simulink model "FullCardioLabModel"  (R2023b)
settings: Solver=FixedStepDiscrete  StartTime=0.0  StopTime=param_sim_time  FixedStep=1/fs  MaxStep=1/fs  RelTol=1e-3
undefined symbols (not defined in the file): analyses, fdesignblkfcn, fs, gcbh, param_tot_samples
libraries: dspstat3 x13, SCGAnalysis_SignalGenerationLib x2
(part 1 of 20)
settings Model: PacingRate=100  Creator=rcord  LastModifiedBy=rcord
settings SolverCC: ZeroCrossControl=DisableAll  AlgebraicLoopSolver=TrustRegion
settings DataIOCC: ExternalInput=[t, signals.ecg.input, signals.scg.input_x, signals.scg.input_y, signals.scg.input_z]  LoadExternalInput=on  SignalLogging=off  DSMLogging=off  SaveTime=off  ReturnWorkspaceOutputs=off  TimeSaveName=t_preprocessing  OutputSaveName=out_preprocessing  LoggingIntervals=[-inf,inf]
settings DebuggingCC: UnconnectedInputMsg=warning  UnconnectedOutputMsg=warning  UnconnectedLineMsg=warning
settings ModelReferenceCC: EnableRefExpFcnMdlSchedulingChecks=on
settings SFSimCC: CustomCodeUndefinedFunction=UseInterfaceOnly
settings RTWCC: DLArmComputeVersion=19.05

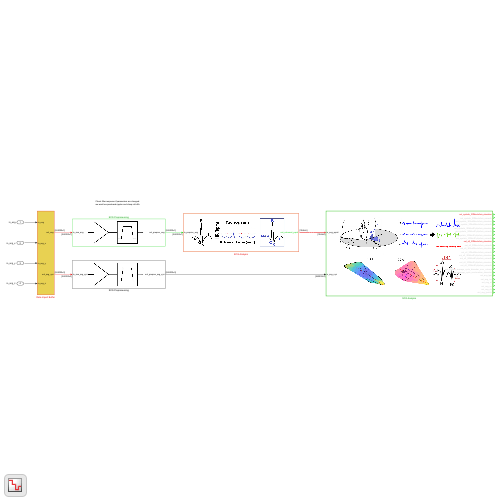
[thumbnail: Simulink's stored preview of the top-level diagram]
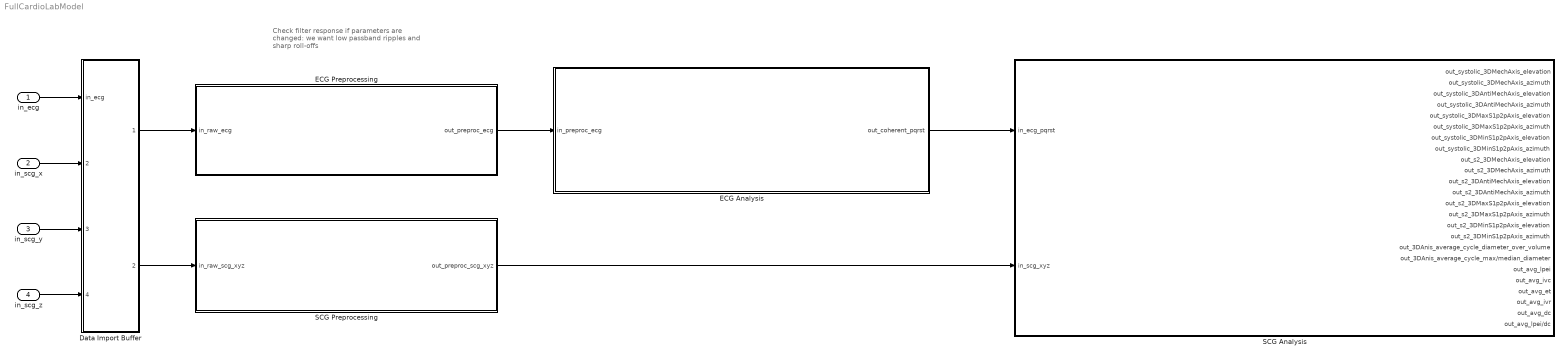
== system FullCardioLabModel ==
  note: Check filter response if parameters are changed:
      | we want low passband ripples and sharp roll-offs
  in_ecg : Inport  SampleTime=1/fs
  in_scg_x : Inport  Port=2  SampleTime=1/fs
  in_scg_y : Inport  Port=3  SampleTime=1/fs
  in_scg_z : Inport  Port=4  SampleTime=1/fs
  Data Import Buffer : Subsystem
  ECG Analysis : Subsystem
      mask Display: image('ECG Analysis2.jpg');
  ECG Preprocessing : Subsystem  mask{param_ecg_gain_mv=1000, param_ecg_fc_lo=1.05, param_ecg_fc_hi=45, param_ecg_trans_bw=1}
      mask prompts: param_ecg_gain_mv "mV Conversion Gain"; param_ecg_fc_lo "Low Passband Frequency Corner (Hz)"; param_ecg_fc_hi "High Passband Frequency Corner (Hz)"; param_ecg_trans_bw "Transition Bandwidth (Hz)"
      mask init:
      | assignin('base','param_ecg_gain_mv',param_ecg_gain_mv)
      | assignin('base','param_ecg_fc_lo',param_ecg_fc_lo)
      | assignin('base','param_ecg_fc_hi',param_ecg_fc_hi)
      | assignin('base','param_ecg_trans_bw',param_ecg_trans_bw)
      mask DialogControl DescGroupVar Prompt: ECG Preprocessing
      mask DialogControl DescTextVar Prompt: Preprocessing stage of the ECG. This involves conversion from V to mV and a filtfilt operation (i.e. a zero-phase FIR filtering) specified by the passband cornerns and transition bandwidth.
      mask Display: image('PreprocessingSymbol.jpg');
  SCG Analysis : Subsystem
      mask Display: image('SCG Analysis.png');
  SCG Preprocessing : Subsystem  mask{param_scg_gain_mg=3333, param_scg_fc_lo=5, param_scg_fc_hi=120, param_scg_trans_bw=2.5}
      mask prompts: param_scg_gain_mg "V to mg Conversion Gain"; param_scg_fc_lo "Low Passband Frequency Corner (Hz)"; param_scg_fc_hi "High Passband Frequency Corner (Hz)"; param_scg_trans_bw "Transition bandwidth"
      mask init:
      | assignin('base','param_scg_gain_mg',param_scg_gain_mg)
      | assignin('base','param_scg_fc_lo',param_scg_fc_lo)
      | assignin('base','param_scg_fc_hi',param_scg_fc_hi)
      | assignin('base','param_scg_trans_bw',param_scg_trans_bw)
      mask DialogControl DescGroupVar Prompt: SCG Preprocessing
      mask DialogControl DescTextVar Prompt: The SCG (x, y, and z) preprocessing block. This involves a V to mg conversion (determined by the transducer sensitivity) and a filtfilt operation. This filtfilt operation consists of a zero-phase FIR front-back filtering that is identical for each of the three cartesian acceleration components and is specified by the passband frequency corners and the transition bandwidth.
      mask Display: image('PreprocessingSymbol.jpg');
  wires:
  in_ecg/1 -> Data Import Buffer/1(in_ecg)
  in_scg_x/1 -> Data Import Buffer/2(in_scg_x)
  in_scg_y/1 -> Data Import Buffer/3(in_scg_y)
  in_scg_z/1 -> Data Import Buffer/4(in_scg_z)
  Data Import Buffer/2(out_scg_xyz) -> SCG Preprocessing/1(in_raw_scg_xyz)
  Data Import Buffer/1(out_ecg) -> ECG Preprocessing/1(in_raw_ecg)
  ECG Preprocessing/1(out_preproc_ecg) -> ECG Analysis/1(in_preproc_ecg)
  SCG Preprocessing/1(out_preproc_scg_xyz) -> SCG Analysis/2(in_scg_xyz)
  ECG Analysis/1(out_coherent_pqrst) -> SCG Analysis/1(in_ecg_pqrst)

== system FullCardioLabModel/Data Import Buffer ==
  in_ecg : Inport
  in_scg_x : Inport  Port=2
  in_scg_y : Inport  Port=3
  in_scg_z : Inport  Port=4
  Buffer{,1..3} (4 alike) : Buffer  N=param_tot_samples  OutputFrames=off
  Vector Concatenate : Concatenate  NumInputs=3  Mode=Multidimensional array  ConcatenateDimension=2
  out_ecg : Outport  VectorParamsAs1DForOutWhenUnconnected=off
  out_scg_xyz : Outport  Port=2  VectorParamsAs1DForOutWhenUnconnected=off
  wires:
  in_ecg/1 -> Buffer1/1
  Buffer/1 -> Vector Concatenate/3  "scg_z"
  Buffer3/1 -> Vector Concatenate/1  "scg_x"
  in_scg_x/1 -> Buffer3/1
  Vector Concatenate/1 -> out_scg_xyz/1
  Buffer1/1 -> out_ecg/1
  Buffer2/1 -> Vector Concatenate/2  "scg_y"
  in_scg_z/1 -> Buffer/1
  in_scg_y/1 -> Buffer2/1

== system FullCardioLabModel/ECG Analysis ==
  in_preproc_ecg : Inport
  Enabled ECG Analysis Subsystem : Subsystem  TreatAsAtomicUnit=on
  out_coherent_pqrst : Outport
  wires:
  in_preproc_ecg/1 -> Enabled ECG Analysis Subsystem/Enable
  Enabled ECG Analysis Subsystem/1(idxs_coherent_pqrst) -> out_coherent_pqrst/1

== system FullCardioLabModel/ECG Preprocessing ==
  in_raw_ecg : Inport
  Enabled ECG Preprocessing Subsystem : Subsystem  TreatAsAtomicUnit=on
  out_preproc_ecg : Outport  VectorParamsAs1DForOutWhenUnconnected=off
  wires:
  Enabled ECG Preprocessing Subsystem/1(Output) -> out_preproc_ecg/1
  in_raw_ecg/1 -> Enabled ECG Preprocessing Subsystem/Enable

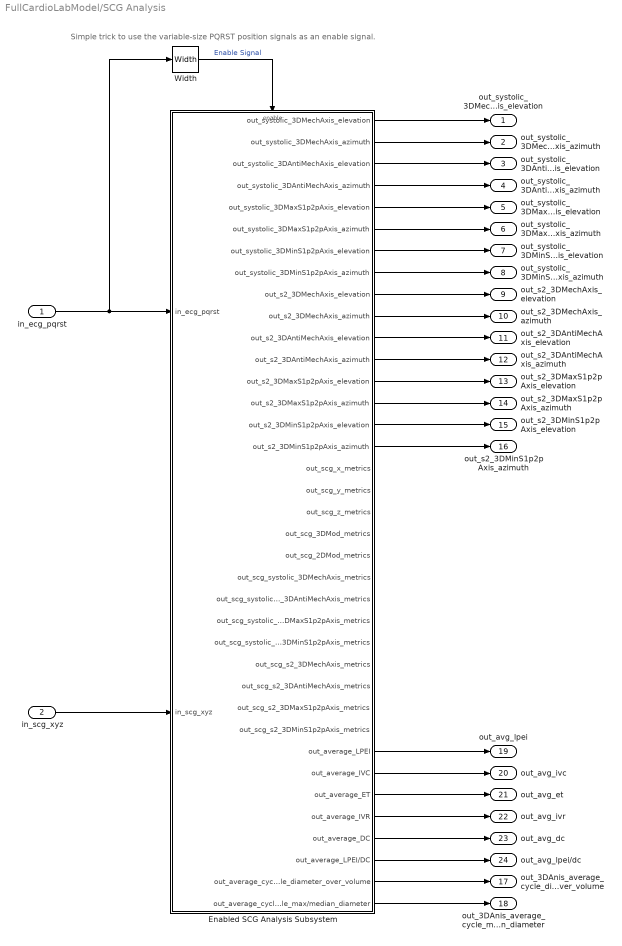
== system FullCardioLabModel/SCG Analysis ==
  note: Simple trick to use the variable-size PQRST position signals as an enable signal.
  in_ecg_pqrst : Inport
  in_scg_xyz : Inport  Port=2
  Enabled SCG Analysis Subsystem : Subsystem  TreatAsAtomicUnit=on
  "Width " : Width
  out_systolic_3DMechAxis_elevation : Outport  VectorParamsAs1DForOutWhenUnconnected=off
  out_systolic_3DMechAxis_azimuth : Outport  Port=2  VectorParamsAs1DForOutWhenUnconnected=off
  out_systolic_3DAntiMechAxis_elevation : Outport  Port=3  VectorParamsAs1DForOutWhenUnconnected=off
  out_systolic_3DAntiMechAxis_azimuth : Outport  Port=4  VectorParamsAs1DForOutWhenUnconnected=off
  out_systolic_3DMaxS1p2pAxis_elevation : Outport  Port=5  VectorParamsAs1DForOutWhenUnconnected=off
  out_systolic_3DMaxS1p2pAxis_azimuth : Outport  Port=6  VectorParamsAs1DForOutWhenUnconnected=off
  out_systolic_3DMinS1p2pAxis_elevation : Outport  Port=7  VectorParamsAs1DForOutWhenUnconnected=off
  out_systolic_3DMinS1p2pAxis_azimuth : Outport  Port=8  VectorParamsAs1DForOutWhenUnconnected=off
  out_s2_3DMechAxis_elevation : Outport  Port=9  VectorParamsAs1DForOutWhenUnconnected=off
  out_s2_3DMechAxis_azimuth : Outport  Port=10  VectorParamsAs1DForOutWhenUnconnected=off
  out_s2_3DAntiMechAxis_elevation : Outport  Port=11  VectorParamsAs1DForOutWhenUnconnected=off
  out_s2_3DAntiMechAxis_azimuth : Outport  Port=12  VectorParamsAs1DForOutWhenUnconnected=off
  out_s2_3DMaxS1p2pAxis_elevation : Outport  Port=13  VectorParamsAs1DForOutWhenUnconnected=off
  out_s2_3DMaxS1p2pAxis_azimuth : Outport  Port=14  VectorParamsAs1DForOutWhenUnconnected=off
  out_s2_3DMinS1p2pAxis_elevation : Outport  Port=15  VectorParamsAs1DForOutWhenUnconnected=off
  out_s2_3DMinS1p2pAxis_azimuth : Outport  Port=16  VectorParamsAs1DForOutWhenUnconnected=off
  out_3DAnis_average_cycle_diameter_over_volume : Outport  Port=17  VectorParamsAs1DForOutWhenUnconnected=off
  out_3DAnis_average_cycle_max/median_diameter : Outport  Port=18  VectorParamsAs1DForOutWhenUnconnected=off
  out_avg_lpei : Outport  Port=19  VectorParamsAs1DForOutWhenUnconnected=off
  out_avg_ivc : Outport  Port=20  VectorParamsAs1DForOutWhenUnconnected=off
  out_avg_et : Outport  Port=21  VectorParamsAs1DForOutWhenUnconnected=off
  out_avg_ivr : Outport  Port=22  VectorParamsAs1DForOutWhenUnconnected=off
  out_avg_dc : Outport  Port=23  VectorParamsAs1DForOutWhenUnconnected=off
  out_avg_lpei/dc : Outport  Port=24  VectorParamsAs1DForOutWhenUnconnected=off
  wires:
  in_scg_xyz/1 -> Enabled SCG Analysis Subsystem/2(in_scg_xyz)
  in_ecg_pqrst/1 -> "Width "/1, Enabled SCG Analysis Subsystem/1(in_ecg_pqrst)
  "Width "/1 -> Enabled SCG Analysis Subsystem/Enable  "Enable Signal"
  Enabled SCG Analysis Subsystem/1(out_systolic_3DMechAxis_elevation) -> out_systolic_3DMechAxis_elevation/1
  Enabled SCG Analysis Subsystem/2(out_systolic_3DMechAxis_azimuth) -> out_systolic_3DMechAxis_azimuth/1
  Enabled SCG Analysis Subsystem/8(out_systolic_3DMinS1p2pAxis_azimuth) -> out_systolic_3DMinS1p2pAxis_azimuth/1
  Enabled SCG Analysis Subsystem/7(out_systolic_3DMinS1p2pAxis_elevation) -> out_systolic_3DMinS1p2pAxis_elevation/1
  Enabled SCG Analysis Subsystem/6(out_systolic_3DMaxS1p2pAxis_azimuth) -> out_systolic_3DMaxS1p2pAxis_azimuth/1
  Enabled SCG Analysis Subsystem/5(out_systolic_3DMaxS1p2pAxis_elevation) -> out_systolic_3DMaxS1p2pAxis_elevation/1
  Enabled SCG Analysis Subsystem/4(out_systolic_3DAntiMechAxis_azimuth) -> out_systolic_3DAntiMechAxis_azimuth/1
  Enabled SCG Analysis Subsystem/3(out_systolic_3DAntiMechAxis_elevation) -> out_systolic_3DAntiMechAxis_elevation/1
  Enabled SCG Analysis Subsystem/37(out_average_cycle_cycle_max/median_diameter) -> out_3DAnis_average_cycle_max/median_diameter/1
  Enabled SCG Analysis Subsystem/36(out_average_cycle_diameter_over_volume) -> out_3DAnis_average_cycle_diameter_over_volume/1
  Enabled SCG Analysis Subsystem/12(out_s2_3DAntiMechAxis_azimuth) -> out_s2_3DAntiMechAxis_azimuth/1
  Enabled SCG Analysis Subsystem/10(out_s2_3DMechAxis_azimuth) -> out_s2_3DMechAxis_azimuth/1
  Enabled SCG Analysis Subsystem/13(out_s2_3DMaxS1p2pAxis_elevation) -> out_s2_3DMaxS1p2pAxis_elevation/1
  Enabled SCG Analysis Subsystem/11(out_s2_3DAntiMechAxis_elevation) -> out_s2_3DAntiMechAxis_elevation/1
  Enabled SCG Analysis Subsystem/14(out_s2_3DMaxS1p2pAxis_azimuth) -> out_s2_3DMaxS1p2pAxis_azimuth/1
  Enabled SCG Analysis Subsystem/15(out_s2_3DMinS1p2pAxis_elevation) -> out_s2_3DMinS1p2pAxis_elevation/1
  Enabled SCG Analysis Subsystem/16(out_s2_3DMinS1p2pAxis_azimuth) -> out_s2_3DMinS1p2pAxis_azimuth/1
  Enabled SCG Analysis Subsystem/9(out_s2_3DMechAxis_elevation) -> out_s2_3DMechAxis_elevation/1
  Enabled SCG Analysis Subsystem/30(out_average_LPEI) -> out_avg_lpei/1
  Enabled SCG Analysis Subsystem/31(out_average_IVC) -> out_avg_ivc/1
  Enabled SCG Analysis Subsystem/32(out_average_ET) -> out_avg_et/1
  Enabled SCG Analysis Subsystem/33(out_average_IVR) -> out_avg_ivr/1
  Enabled SCG Analysis Subsystem/34(out_average_DC) -> out_avg_dc/1
  Enabled SCG Analysis Subsystem/35(out_average_LPEI/DC) -> out_avg_lpei/dc/1

== system FullCardioLabModel/SCG Preprocessing ==
  in_raw_scg_xyz : Inport
  Enabled SCG Preprocessing Subsystem : Subsystem  TreatAsAtomicUnit=on
  out_preproc_scg_xyz : Outport  VectorParamsAs1DForOutWhenUnconnected=off
  wires:
  Enabled SCG Preprocessing Subsystem/1(out_preprocessed_scg_xyz) -> out_preproc_scg_xyz/1
  in_raw_scg_xyz/1 -> Enabled SCG Preprocessing Subsystem/Enable

== system FullCardioLabModel/ECG Analysis/Enabled ECG Analysis Subsystem ==
  note: The subsystem is only enabled when it receives a (non-zero) signal
  Preprocessed ECG : EnablePort  PropagateVarSize=During execution  ShowOutputPort=on
  Assign To Workspace: Num Cycles : Subsystem
      mask Display: disp('Assign: out_ecg_num_cycles')
  Assign To Workspace: idxs PQRST : Subsystem
      mask Display: disp('Assign: out_idxs_pqrst')
  Coherent Segmentation : Subsystem
      mask Display: image('Coherent ECG.jpg');
  Constant : Constant  Value=fs
  Ectopic Correction : Subsystem  mask{max_hr=200, max_hr_dev=40}
      mask prompts: max_hr "Maximum Heart Rate (in bpm)"; max_hr_dev "Maximum HR Deviation (in bpm)"
      mask DialogControl DescGroupVar Prompt: Ectopic Correction
      mask DialogControl DescTextVar Prompt: Specify the ectopic detection parameters. What will be defined as an ectopic cycle and removed from further analysis? Maximum heart rate specifies the upper limit of heart rate - any cycles with RR intervals corresponding to heart rates above this limit will be considered ectopic. Maximum HR deviation - any cycles with an instantaneous HR greater than this deviation from the moving average HR will be considered ectopic.
      mask Display: image('Tachogram.jpg');
  Labelled ECG Plotting : MATLAB Function  TreatAsAtomicUnit=on
  Num Cycles : Display
  P,Q,R,S,T Detection : Subsystem  mask{ecg_algo=PQRST waves - Multi-level Teager Energy Operator}
      mask prompts: ecg_algo "Choose one:"
      mask init:
      | if ecg_algo == 1
      |     param_ecg_algo = 'Pan-Tompkins';
      | elseif ecg_algo == 2
      |     param_ecg_algo = 'Phase Space';
      | elseif ecg_algo == 3
      |     param_ecg_algo = 'Filter Bank';
      | elseif ecg_algo == 4
      |     param_ecg_algo = 'State Machine';
      | elseif ecg_algo == 5
      |     param_ecg_algo = 'Multi-level Teager Energy Operator';
      | end
      | 
      | assignin('base','param_ecg_algo', param_ecg_algo)
      mask TypeOptions ecg_algo: R wave  - Pan-Tompkins | R wave - Phase space | R wave - Filter bank | QRST waves - State machine | PQRST waves - Multi-level Teager Energy Operator
      mask DialogControl DescGroupVar Prompt: ECG PQRST Detection
      mask DialogControl DescTextVar Prompt: Select detected waveform(s) and corresponding detection aglorithm.
      mask DialogControl ParameterGroupVar Prompt: Desired wave(s) and Algorithm
      mask Display: image('Labelled ECG2.jpg');
  idxs_coherent_pqrst : Outport
  wires:
  Preprocessed ECG/1 -> P,Q,R,S,T Detection/1(Preprocessed ECG), Labelled ECG Plotting/2(preprocessed_ecg)
  P,Q,R,S,T Detection/3(idxs_r) -> Ectopic Correction/1(r_pos)
  Constant/1 -> Labelled ECG Plotting/3(fs)
  Coherent Segmentation/2(num_cycles) -> Assign To Workspace: Num Cycles/1(In1), Num Cycles/1
  Ectopic Correction/1(corrected_r_pos) -> Coherent Segmentation/3(idxs_r)
  Coherent Segmentation/1(idxs_coherent_pqrst) -> Assign To Workspace: idxs PQRST/1(in_idxs_pqrst), idxs_coherent_pqrst/1, Labelled ECG Plotting/1(idxs_coherent_pqrst)
  P,Q,R,S,T Detection/5(idxs_t) -> Coherent Segmentation/5(idxs_t)
  P,Q,R,S,T Detection/4(idxs_s) -> Coherent Segmentation/4(idxs_s)
  P,Q,R,S,T Detection/1(idxs_p) -> Coherent Segmentation/1(idxs_p)
  P,Q,R,S,T Detection/2(idxs_q) -> Coherent Segmentation/2(idxs_q)

== system FullCardioLabModel/ECG Preprocessing/Enabled ECG Preprocessing Subsystem ==
  note: The subsystem is only enabled when it receives a (non-zero) signal
  in_ecg : EnablePort  ShowOutputPort=on
  Constant : Constant  Value=fs
  ECG Filtfiltering : Subsystem
  ECG Preprocessing Input (Frequency) : SpectrumAnalyzer  Commented=on  WindowPosition=[1 1 1312 537]  Method=Welch  SampleRate=1000  PlotAsTwoSidedSpectrum=off  Span=500  CenterFrequency=250  StartFrequency=0  StopFrequency=500  FrequencyResolutionMethod=Window length  WindowLength=param_tot_samples/10  Window=Rectangular  AveragingMethod=Running  SpectralAverages=10  YLimits=[-135.30878679633289607,-53.597859807423823497]  ShowLegend=on  DefaultConfigurationName=spbscopes.SpectrumAnalyzerBlockCfg  IsFrequencyInputMode=0  FrequencyVectorPort=0  FrequencyVectorFromPort=0  FrequencyInputRBWPort=0  FrequencyInputRBWFromPort=0
  ECG Preprocessing Input (Time) : Scope  Commented=on
  ECG Preprocessing Output (Frequency) : SpectrumAnalyzer  Commented=on  WindowPosition=[1 1 1312 537]  Method=Welch  SampleRateSource=Property  SampleRate=1/fs  PlotAsTwoSidedSpectrum=off  Span=0.0005  CenterFrequency=0.00025  StartFrequency=0  StopFrequency=0.0005  FrequencyResolutionMethod=Window length  WindowLength=param_tot_samples/10  Window=Rectangular  AveragingMethod=Running  SpectralAverages=10  YLimits=[-88.467038023731845442,-3.7161177694563978235]  ShowLegend=on  DefaultConfigurationName=spbscopes.SpectrumAnalyzerBlockCfg  IsFrequencyInputMode=0  FrequencyVectorPort=0  FrequencyVectorFromPort=0  FrequencyInputRBWPort=0  FrequencyInputRBWFromPort=0
  ECG Preprocessing Output (Time) : Scope
  Plotting : MATLAB Function  TreatAsAtomicUnit=on
  To Workspace: Processed ECG : Subsystem
      mask Display: disp('out_ecg_preprocessing')
  V to mV Conversion : Gain  Gain=param_ecg_gain_mv
  Output : Outport  VectorParamsAs1DForOutWhenUnconnected=off
  wires:
  V to mV Conversion/1 -> ECG Filtfiltering/1(input ecg)
  in_ecg/1 -> V to mV Conversion/1, ECG Preprocessing Input (Time)/1, Plotting/2(raw_ecg), ECG Preprocessing Input (Frequency)/1
  ECG Filtfiltering/1(filtfiltered ecg) -> To Workspace: Processed ECG/1(In1), Output/1, ECG Preprocessing Output (Time)/1, Plotting/1(preprocessed_ecg), ECG Preprocessing Output (Frequency)/1
  Constant/1 -> Plotting/3(fs)

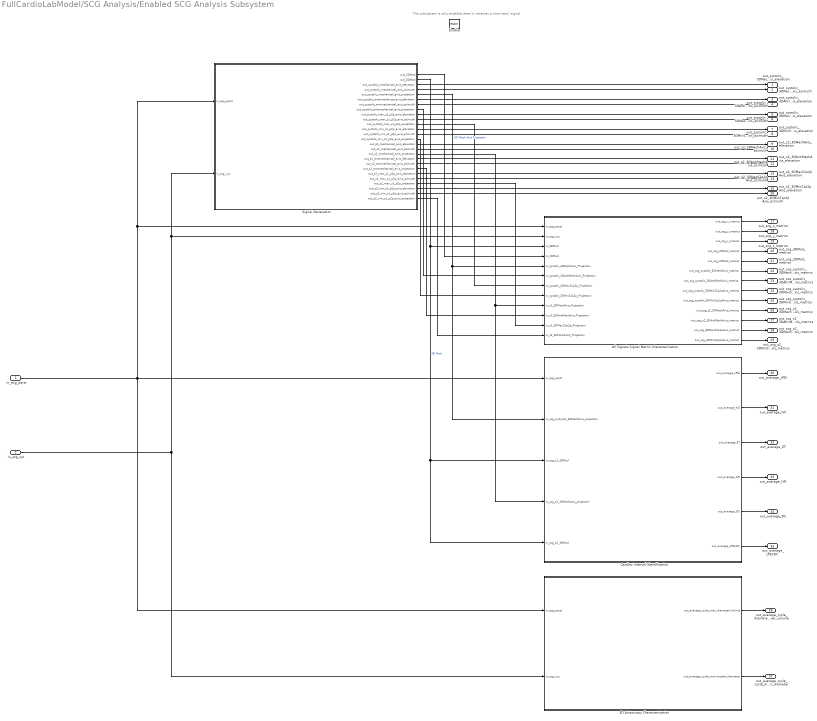
== system FullCardioLabModel/SCG Analysis/Enabled SCG Analysis Subsystem ==
  note: The subsystem is only enabled when it receives a (non-zero) signal
  in_ecg_pqrst : Inport
  in_scg_xyz : Inport  Port=2
  Enable : EnablePort  StatesWhenEnabling=reset  PropagateVarSize=During execution
  3D Anisotropy Characterization : Subsystem
      mask Display: image('Anisotropy.png');
  All Signals Signal Metric Characterization : Subsystem
      mask Display: image('Characterization.png');
  Cardiac Interval Identification : Subsystem
      mask Display: image('Systolic Intervals.png');
  Signal Generation : Subsystem
      mask Display: image('Signal Generation.png');
  out_systolic_3DMechAxis_elevation : Outport  VectorParamsAs1DForOutWhenUnconnected=off
  out_systolic_3DMechAxis_azimuth : Outport  Port=2  VectorParamsAs1DForOutWhenUnconnected=off
  out_systolic_3DAntiMechAxis_elevation : Outport  Port=3  VectorParamsAs1DForOutWhenUnconnected=off
  out_systolic_3DAntiMechAxis_azimuth : Outport  Port=4  VectorParamsAs1DForOutWhenUnconnected=off
  out_systolic_3DMaxS1p2pAxis_elevation : Outport  Port=5  VectorParamsAs1DForOutWhenUnconnected=off
  out_systolic_3DMaxS1p2pAxis_azimuth : Outport  Port=6  VectorParamsAs1DForOutWhenUnconnected=off
  out_systolic_3DMinS1p2pAxis_elevation : Outport  Port=7  VectorParamsAs1DForOutWhenUnconnected=off
  out_systolic_3DMinS1p2pAxis_azimuth : Outport  Port=8  VectorParamsAs1DForOutWhenUnconnected=off
  out_s2_3DMechAxis_elevation : Outport  Port=9  VectorParamsAs1DForOutWhenUnconnected=off
  out_s2_3DMechAxis_azimuth : Outport  Port=10  VectorParamsAs1DForOutWhenUnconnected=off
  out_s2_3DAntiMechAxis_elevation : Outport  Port=11  VectorParamsAs1DForOutWhenUnconnected=off
  out_s2_3DAntiMechAxis_azimuth : Outport  Port=12  VectorParamsAs1DForOutWhenUnconnected=off
  out_s2_3DMaxS1p2pAxis_elevation : Outport  Port=13  VectorParamsAs1DForOutWhenUnconnected=off
  out_s2_3DMaxS1p2pAxis_azimuth : Outport  Port=14  VectorParamsAs1DForOutWhenUnconnected=off
  out_s2_3DMinS1p2pAxis_elevation : Outport  Port=15  VectorParamsAs1DForOutWhenUnconnected=off
  out_s2_3DMinS1p2pAxis_azimuth : Outport  Port=16  VectorParamsAs1DForOutWhenUnconnected=off
  out_scg_x_metrics : Outport  Port=17
  out_scg_y_metrics : Outport  Port=18
  out_scg_z_metrics : Outport  Port=19
  out_scg_3DMod_metrics : Outport  Port=20
  out_scg_2DMod_metrics : Outport  Port=21
  out_scg_systolic_3DMechAxis_metrics : Outport  Port=22
  out_scg_systolic_3DAntiMechAxis_metrics : Outport  Port=23
  out_scg_systolic_3DMaxS1p2pAxis_metrics : Outport  Port=24
  out_scg_systolic_3DMinS1p2pAxis_metrics : Outport  Port=25
  out_scg_s2_3DMechAxis_metrics : Outport  Port=26
  out_scg_s2_3DAntiMechAxis_metrics : Outport  Port=27
  out_scg_s2_3DMaxS1p2pAxis_metrics : Outport  Port=28
  out_scg_s2_3DMinS1p2pAxis_metrics : Outport  Port=29
  out_average_LPEI : Outport  Port=30
  out_average_IVC : Outport  Port=31
  out_average_ET : Outport  Port=32
  out_average_IVR : Outport  Port=33
  out_average_DC : Outport  Port=34
  out_average_LPEI/DC : Outport  Port=35
  out_average_cycle_diameter_over_volume : Outport  Port=36  VectorParamsAs1DForOutWhenUnconnected=off
  out_average_cycle_cycle_max/median_diameter : Outport  Port=37  VectorParamsAs1DForOutWhenUnconnected=off
  wires:
  Signal Generation/1(out_2DMod) -> All Signals Signal Metric Characterization/4(in_2DMod)
  Signal Generation/2(out_3DMod) -> Cardiac Interval Identification/3(in_scg_s1_3DMod), Cardiac Interval Identification/5(in_scg_s2_3DMod), All Signals Signal Metric Characterization/3(in_3DMod)  "3D Mod"
  in_scg_xyz/1 -> 3D Anisotropy Characterization/2(in_scg_xyz), Signal Generation/2(in_scg_xyz), All Signals Signal Metric Characterization/2(in_scg_xyz)
  in_ecg_pqrst/1 -> Signal Generation/1(in_ecg_pqrst), All Signals Signal Metric Characterization/1(in_ecg_pqrst), 3D Anisotropy Characterization/1(in_ecg_pqrst), Cardiac Interval Identification/1(in_ecg_pqrst)
  Signal Generation/3(out_systolic_mechanical_axis_elevation) -> out_systolic_3DMechAxis_elevation/1
  Signal Generation/4(out_systolic_mechanical_axis_azimuth) -> out_systolic_3DMechAxis_azimuth/1
  Signal Generation/5(out_systolic_mechanical_axis_projection) -> Cardiac Interval Identification/2(in_scg_systyolic_3DMechAxis_projection), All Signals Signal Metric Characterization/5(in_systolic_3DMechAxis_Projection)  "3D Mech Axis Projection"
  Signal Generation/6(out_systolic_antimechanical_axis_elevation) -> out_systolic_3DAntiMechAxis_elevation/1
  Signal Generation/7(out_systolic_antimechanical_axis_azimuth) -> out_systolic_3DAntiMechAxis_azimuth/1
  Signal Generation/8(out_systolic_antimechanical_axis_projection) -> All Signals Signal Metric Characterization/6(in_systolic_3DAntiMechAxis_Projection)
  Signal Generation/9(out_systolic_max_s1_p2p_axis_elevation) -> out_systolic_3DMaxS1p2pAxis_elevation/1
  Signal Generation/10(out_systolic_max_s1_p2p_axis_azimuth) -> out_systolic_3DMaxS1p2pAxis_azimuth/1
  Signal Generation/11(out_systolic_max_s1_p2p_projection) -> All Signals Signal Metric Characterization/7(in_systolic_3DMaxS1p2p_Projection)
  Signal Generation/12(out_systolic_min_s1_p2p_axis_elevation) -> out_systolic_3DMinS1p2pAxis_elevation/1
  Signal Generation/13(out_systolic_min_s1_p2p_axis_azimuth) -> out_systolic_3DMinS1p2pAxis_azimuth/1
  Signal Generation/14(out_systolic_min_s1_p2p_axis_projection) -> All Signals Signal Metric Characterization/8(in_systolic_3DMinS1p2p_Projection)
  3D Anisotropy Characterization/1(out_average_cycle_max_diameter/volume) -> out_average_cycle_diameter_over_volume/1
  3D Anisotropy Characterization/2(out_average_cycle_max/median_diameter) -> out_average_cycle_cycle_max/median_diameter/1
  All Signals Signal Metric Characterization/1(out_scg_x_metrics) -> out_scg_x_metrics/1
  All Signals Signal Metric Characterization/2(out_scg_y_metrics) -> out_scg_y_metrics/1
  All Signals Signal Metric Characterization/3(out_scg_z_metrics) -> out_scg_z_metrics/1
  All Signals Signal Metric Characterization/4(out_scg_3DMod_metrics) -> out_scg_3DMod_metrics/1
  All Signals Signal Metric Characterization/5(out_scg_2DMod_metrics) -> out_scg_2DMod_metrics/1
  All Signals Signal Metric Characterization/6(out_scg_systolic_3DMechAxis_metrics) -> out_scg_systolic_3DMechAxis_metrics/1
  All Signals Signal Metric Characterization/7(out_scg_systolic_3DAntiMechAxis_metrics) -> out_scg_systolic_3DAntiMechAxis_metrics/1
  All Signals Signal Metric Characterization/8(out_scg_systolic_3DMaxS1p2pAxis_metrics) -> out_scg_systolic_3DMaxS1p2pAxis_metrics/1
  All Signals Signal Metric Characterization/9(out_scg_systolic_3DMinS1p2pAxis_metrics) -> out_scg_systolic_3DMinS1p2pAxis_metrics/1
  Signal Generation/15(out_s2_mechanical_axis_elevation) -> out_s2_3DMechAxis_elevation/1
  Signal Generation/16(out_s2_mechanical_axis_azimuth) -> out_s2_3DMechAxis_azimuth/1
  Signal Generation/17(out_s2_mechanical_axis_projection) -> Cardiac Interval Identification/4(in_scg_s2_3DMechAxis_projection), All Signals Signal Metric Characterization/9(in_s2_3DMechAxis_Projection)
  Signal Generation/18(out_s2_antimechanical_axis_elevation) -> out_s2_3DAntiMechAxis_elevation/1
  Signal Generation/19(out_s2_antimechanical_axis_azimuth) -> out_s2_3DAntiMechAxis_azimuth/1
  Signal Generation/20(out_s2_antimechanical_axis_projection) -> All Signals Signal Metric Characterization/10(in_s2_3DAntiMechAxis_Projection)
  Signal Generation/21(out_s2_max_s1_p2p_axis_elevation) -> out_s2_3DMaxS1p2pAxis_elevation/1
  Signal Generation/22(out_s2_max_s1_p2p_axis_azimuth) -> out_s2_3DMaxS1p2pAxis_azimuth/1
  Signal Generation/23(out_s2_max_s1_p2p_projection) -> All Signals Signal Metric Characterization/11(in_s2_3DMaxS1p2p_Projection)
  Signal Generation/24(out_s2_min_s1_p2p_axis_elevation) -> out_s2_3DMinS1p2pAxis_elevation/1
  Signal Generation/26(out_s2_min_s1_p2p_axis_projection) -> All Signals Signal Metric Characterization/12(in_s2_3DMinS1p2p_Projection)
  Signal Generation/25(out_s2_min_s1_p2p_axis_azimuth) -> out_s2_3DMinS1p2pAxis_azimuth/1
  All Signals Signal Metric Characterization/13(out_scg_3DMinS2p2pAxis_metrics) -> out_scg_s2_3DMinS1p2pAxis_metrics/1
  All Signals Signal Metric Characterization/12(out_scg_3DMaxS2p2pAxis_metrics) -> out_scg_s2_3DMaxS1p2pAxis_metrics/1
  All Signals Signal Metric Characterization/10(out_scg_s2_3DMechAxis_metrics) -> out_scg_s2_3DMechAxis_metrics/1
  All Signals Signal Metric Characterization/11(out_scg_s2_3DAntiMechAxis_metrics) -> out_scg_s2_3DAntiMechAxis_metrics/1
  Cardiac Interval Identification/1(out_average_LPEI) -> out_average_LPEI/1
  Cardiac Interval Identification/2(out_average_IVC) -> out_average_IVC/1
  Cardiac Interval Identification/3(out_average_ET) -> out_average_ET/1
  Cardiac Interval Identification/4(out_average_IVR) -> out_average_IVR/1
  Cardiac Interval Identification/5(out_average_DC) -> out_average_DC/1
  Cardiac Interval Identification/6(out_average_LPEI/DC) -> out_average_LPEI/DC/1

== system FullCardioLabModel/SCG Preprocessing/Enabled SCG Preprocessing Subsystem ==
  note: The subsystem is only enabled when it receives a (non-zero) signal
  in_scg_xyz : EnablePort  ShowOutputPort=on
  Constant : Constant  Value=fs
  Filtfiltering : Subsystem
  Plotting : MATLAB Function  TreatAsAtomicUnit=on
  SCG Preprocessing Input (Frequency) : SpectrumAnalyzer  Commented=on  WindowPosition=[1 1 1312 537]  Method=Welch  SampleRate=1000  PlotAsTwoSidedSpectrum=off  Span=500  CenterFrequency=250  StartFrequency=0  StopFrequency=500  FrequencyResolutionMethod=Window length  WindowLength=param_tot_samples/10  Window=Rectangular  AveragingMethod=Running  SpectralAverages=10  YLimits=[-95.620326188963844061,-23.201044461318168999]  ShowLegend=on  DefaultConfigurationName=spbscopes.SpectrumAnalyzerBlockCfg  IsFrequencyInputMode=0  FrequencyVectorPort=0  FrequencyVectorFromPort=0  FrequencyInputRBWPort=0  FrequencyInputRBWFromPort=0
  SCG Preprocessing Input (Time) : Scope  Commented=on
  SCG Preprocessing Output (Frequency) : SpectrumAnalyzer  Commented=on  WindowPosition=[1 1 1312 537]  Method=Welch  SampleRate=1000  PlotAsTwoSidedSpectrum=off  AxesScaling=Manual  Span=500  CenterFrequency=250  StartFrequency=0  StopFrequency=500  FrequencyResolutionMethod=Window length  WindowLength=param_tot_samples/10  Window=Rectangular  AveragingMethod=Running  SpectralAverages=10  YLimits=[-56.189595382211429353,39.464899614417547014]  ShowLegend=on  DefaultConfigurationName=spbscopes.SpectrumAnalyzerBlockCfg  IsFrequencyInputMode=0  FrequencyVectorPort=0  FrequencyVectorFromPort=0  FrequencyInputRBWPort=0  FrequencyInputRBWFromPort=0
  SCG Preprocessing Output (Time) : Scope  Commented=on
  To Workspace: Processed SCGxyz : Subsystem
      mask Display: disp('out_scg_xyz_preprocessing')
  V to mg Conversion : Gain  Gain=param_scg_gain_mg
  out_preprocessed_scg_xyz : Outport  VectorParamsAs1DForOutWhenUnconnected=off
  wires:
  V to mg Conversion/1 -> Filtfiltering/1(" input SCG")
  Filtfiltering/1(filtfiltered SCG) -> out_preprocessed_scg_xyz/1, To Workspace: Processed SCGxyz/1(In1), Plotting/1(preprocessed_scg_xyz), SCG Preprocessing Output (Frequency)/1, SCG Preprocessing Output (Time)/1
  Constant/1 -> Plotting/3(fs)
  in_scg_xyz/1 -> V to mg Conversion/1, Plotting/2(raw_scg_xyz), SCG Preprocessing Input (Frequency)/1, SCG Preprocessing Input (Time)/1

== system FullCardioLabModel/ECG Analysis/Enabled ECG Analysis Subsystem/Assign To Workspace: Num Cycles ==
  In1 : Inport
  Enabled To Workspace ECG Num Cycles : Subsystem  TreatAsAtomicUnit=on
  wires:
  In1/1 -> Enabled To Workspace ECG Num Cycles/Enable

== system FullCardioLabModel/ECG Analysis/Enabled ECG Analysis Subsystem/Assign To Workspace: idxs PQRST ==
  in_idxs_pqrst : Inport
  Enable Selector : Selector  NumberOfDimensions=2  InputPortWidth=3  IndexOptions=Index vector (dialog),Index vector (dialog)  Indices=[1],[3]  OutputSizes=1,1
  Enabled To Workspace idxs PQRST : Subsystem  TreatAsAtomicUnit=on
  wires:
  in_idxs_pqrst/1 -> Enable Selector/1, Enabled To Workspace idxs PQRST/1(in_idxs_pqrst)
  Enable Selector/1 -> Enabled To Workspace idxs PQRST/Enable  "Enable"

== system FullCardioLabModel/ECG Analysis/Enabled ECG Analysis Subsystem/Coherent Segmentation ==
  note: This selector gets rid of the nan's after the detected cycles.
  idxs_p : Inport
  idxs_q : Inport  Port=2
  idxs_r : Inport  Port=3
  idxs_s : Inport  Port=4
  idxs_t : Inport  Port=5
  Constant : Constant
  Mux : Mux  Inputs=2
  Selector : Selector  NumberOfDimensions=2  InputPortWidth=3  IndexOptions=Starting and ending indices (port),Index vector (dialog)  Indices=[1 3],[1 2 3 3 5]  OutputSizes=1,1
  Slk Coherent Segmentation Function : MATLAB Function  TreatAsAtomicUnit=on
  idxs_coherent_pqrst : Outport
  num_cycles : Outport  Port=2
  wires:
  idxs_q/1 -> Slk Coherent Segmentation Function/2(idxs_q)
  idxs_s/1 -> Slk Coherent Segmentation Function/4(idxs_s)
  idxs_p/1 -> Slk Coherent Segmentation Function/1(idxs_p)
  idxs_r/1 -> Slk Coherent Segmentation Function/3(idxs_r)
  idxs_t/1 -> Slk Coherent Segmentation Function/5(idxs_t)
  Constant/1 -> Mux/1
  Mux/1 -> Selector/2
  Slk Coherent Segmentation Function/1(idxs_coherent_pqrst) -> Selector/1
  Selector/1 -> idxs_coherent_pqrst/1
  Slk Coherent Segmentation Function/2(num_cycles) -> num_cycles/1, Mux/2

== system FullCardioLabModel/ECG Analysis/Enabled ECG Analysis Subsystem/Ectopic Correction ==
  r_pos : Inport
  Constant : Constant  Value=max_hr
  Constant1 : Constant  Value=max_hr_dev
  Constant2 : Constant  Value=fs
  Ectopic Correction : MATLAB Function  TreatAsAtomicUnit=on
  corrected_r_pos : Outport
  wires:
  Ectopic Correction/1(idxs_corrected_r) -> corrected_r_pos/1
  Constant2/1 -> Ectopic Correction/1(fs)
  Constant/1 -> Ectopic Correction/2(max_hr)
  Constant1/1 -> Ectopic Correction/3(max_hr_dev)
  r_pos/1 -> Ectopic Correction/4(idxs_r)

== system FullCardioLabModel/ECG Analysis/Enabled ECG Analysis Subsystem/P,Q,R,S,T Detection ==
  Preprocessed ECG : Inport
  Constant : Constant  Value=fs
  Constant1 : Constant  Value=ecg_algo
  Wrapped BioSigKit ECG PQRST Detection : MATLAB Function  TreatAsAtomicUnit=on
  idxs_p : Outport
      settings: VarSizeSig=Yes
  idxs_q : Outport  Port=2
      settings: VarSizeSig=Yes
  idxs_r : Outport  Port=3
      settings: VarSizeSig=Yes
  idxs_s : Outport  Port=4
      settings: VarSizeSig=Yes
  idxs_t : Outport  Port=5
      settings: VarSizeSig=Yes
  wires:
  Preprocessed ECG/1 -> Wrapped BioSigKit ECG PQRST Detection/2(preprocessed_ecg)
  Constant/1 -> Wrapped BioSigKit ECG PQRST Detection/1(fs)
  Wrapped BioSigKit ECG PQRST Detection/1(idxs_p) -> idxs_p/1
  Wrapped BioSigKit ECG PQRST Detection/2(idxs_q) -> idxs_q/1
  Wrapped BioSigKit ECG PQRST Detection/3(idxs_r) -> idxs_r/1
  Wrapped BioSigKit ECG PQRST Detection/4(idxs_s) -> idxs_s/1
  Wrapped BioSigKit ECG PQRST Detection/5(idxs_t) -> idxs_t/1
  Constant1/1 -> Wrapped BioSigKit ECG PQRST Detection/3(ecg_algo)

== system FullCardioLabModel/ECG Preprocessing/Enabled ECG Preprocessing Subsystem/ECG Filtfiltering ==
  input ecg : Inport
  Bandpass Filter 1 : Subsystem  DialogController=fdesignblkfcn  InitFcn=fdesignblkfcn(gcbh, {'InitFcn'});  mask(Bandpass Filter){}
      mask help: Design a bandpass filter
      settings: CopyFcn=fdesignblkfcn(gcbh, {'CopyFcn'});
      mask Help: helpview(mapfilelocation('dsp'), 'dspbandpassfilter');
      mask Display: disp('Bandpass');
  Bandpass Filter 2 : Subsystem  DialogController=fdesignblkfcn  InitFcn=fdesignblkfcn(gcbh, {'InitFcn'});  mask(Bandpass Filter){}
      mask help: Design a bandpass filter
      settings: CopyFcn=fdesignblkfcn(gcbh, {'CopyFcn'});
      mask Help: helpview(mapfilelocation('dsp'), 'dspbandpassfilter');
      mask Display: disp('Bandpass');
  Flip : DSPFlip
  Flip1 : DSPFlip
  filtfiltered ecg : Outport  VectorParamsAs1DForOutWhenUnconnected=off
  wires:
  Flip/1 -> Bandpass Filter 2/1(In)
  input ecg/1 -> Bandpass Filter 1/1(In)
  Flip1/1 -> filtfiltered ecg/1
  Bandpass Filter 1/1(Out) -> Flip/1
  Bandpass Filter 2/1(Out) -> Flip1/1

== system FullCardioLabModel/ECG Preprocessing/Enabled ECG Preprocessing Subsystem/To Workspace: Processed ECG ==
  In1 : Inport
  Enabled To Workspace ECG Subsystem : Subsystem  TreatAsAtomicUnit=on
  wires:
  In1/1 -> Enabled To Workspace ECG Subsystem/Enable, Enabled To Workspace ECG Subsystem/1(In1)

== system FullCardioLabModel/SCG Analysis/Enabled SCG Analysis Subsystem/3D Anisotropy Characterization ==
  in_ecg_pqrst : Inport
  in_scg_xyz : Inport  Port=2
  Average Cycle Max Diameter/Volume Calculator : Subsystem
  Average Cycle Max/Median Diameter Calculator : Subsystem
  Display2 : Display
  Display6 : Display
  R Wave Selector : Selector  NumberOfDimensions=2  InputPortWidth=3  IndexOptions=Select all,Index vector (dialog)  Indices=[1 3],3  OutputSizes=1,1
  out_average_cycle_max_diameter/volume : Outport
  out_average_cycle_max/median_diameter : Outport  Port=2
  wires:
  in_ecg_pqrst/1 -> R Wave Selector/1
  in_scg_xyz/1 -> Average Cycle Max Diameter/Volume Calculator/2(in_scg_xyz), Average Cycle Max/Median Diameter Calculator/2(in_scg_xyz)
  Average Cycle Max Diameter/Volume Calculator/1(out_average_cycle_max_diameter/volume) -> Display2/1, out_average_cycle_max_diameter/volume/1
  R Wave Selector/1 -> Average Cycle Max Diameter/Volume Calculator/1(in_r_pos), Average Cycle Max/Median Diameter Calculator/1(in_r_pos)  "R pos"
  Average Cycle Max/Median Diameter Calculator/1(out_average_cycle_max/median_diameter) -> out_average_cycle_max/median_diameter/1, Display6/1
